simulink model "bad_idea"  (Simulink 4.00)
settings: Solver=FixedStepDiscrete  StartTime=0.0  StopTime=inf  FixedStep=Ts  RelTol=1e-3
values from neighbouring files (symbols this model uses):
  Ts = 5e-3    (= 0.005)    [makeplant.m]    (also in profile3.m = acc; recalc.m = 0.001)
libraries: motion x3, simulink3 x1
settings Model: LastModifiedBy=plambrec  SaveTime=off  MaxDataPoints=10000  BlockReductionOpt=off

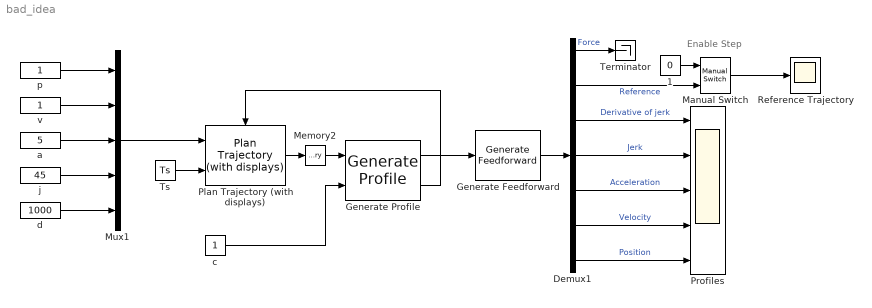
== system bad_idea ==
  note: Enable Step
  1 : Constant  Value=0
  Demux1 : Demux  Outputs=7  BusSelectionMode=off
  Generate Feedforward : motion/Real Time/Generate Feedforward  m1=20  m2=10  k1=10  k2=10  c=6e5  k12=500  Ts=Ts  S1=1  S2=1
  Generate Profile : motion/Real Time/Generate Profile  Ts=Ts  Tset=1  Sdir=1
  Manual Switch : simulink3/Nonlinear/Manual Switch  sw=0  action=0
  Memory2 : Memory  X0=0  InheritSampleTime=on
  Mux1 : Mux  Inputs=5
  Plan Trajectory (with displays) : motion/Real Time/Plan Trajectory (with displays)  TreatAsAtomicUnit=on
      settings: RTWFcnNameOpts=Auto  RTWFileNameOpts=Auto
  Profiles : Scope  NumInputPorts=5
      settings: TimeRange=50  YMin=-1000~-50~-5~-1~-0.5  YMax=1000~50~5~1~1  SaveToWorkspace=off  SaveName=ScopeData2  LimitDataPoints=on  MaxDataPoints=50000
  Reference Trajectory : Scope
      settings: TimeRange=3  YMin=-0.2  YMax=1.2  SaveToWorkspace=off  LimitDataPoints=on  MaxDataPoints=50000
  Terminator : Terminator
  Ts : Constant  Value=Ts
  a : Constant  Value=5
  c : Constant  Value=1
  d : Constant  Value=1000
  j : Constant  Value=45
  p : Constant  Value=1
  v : Constant  Value=1
  wires:
  v/1 -> Mux1/2
  a/1 -> Mux1/3
  j/1 -> Mux1/4
  d/1 -> Mux1/5
  p/1 -> Mux1/1
  Demux1/3 -> Profiles/1  "Derivative of jerk"
  Demux1/4 -> Profiles/2  "Jerk"
  Demux1/5 -> Profiles/3  "Acceleration"
  Demux1/6 -> Profiles/4  "Velocity"
  Demux1/7 -> Profiles/5  "Position"
  Plan Trajectory (with displays)/1 -> Memory2/1
  Memory2/1 -> Generate Profile/1
  Generate Profile/2 -> Plan Trajectory (with displays)/Trigger
  Generate Profile/1 -> Generate Feedforward/1
  Generate Feedforward/1 -> Demux1/1
  c/1 -> Generate Profile/2
  Mux1/1 -> Plan Trajectory (with displays)/1
  Ts/1 -> Plan Trajectory (with displays)/2
  Demux1/2 -> Manual Switch/2  "Reference"
  1/1 -> Manual Switch/1
  Manual Switch/1 -> Reference Trajectory/1
  Demux1/1 -> Terminator/1  "Force"
